simulink library "Fil"  (R2013b)
settings: Solver=ode45  StartTime=0.0  StopTime=10.0  RelTol=1e-3
libraries: Fil x5
settings Model: Creator=qzwc4r  LastModifiedBy=DZ1YRM

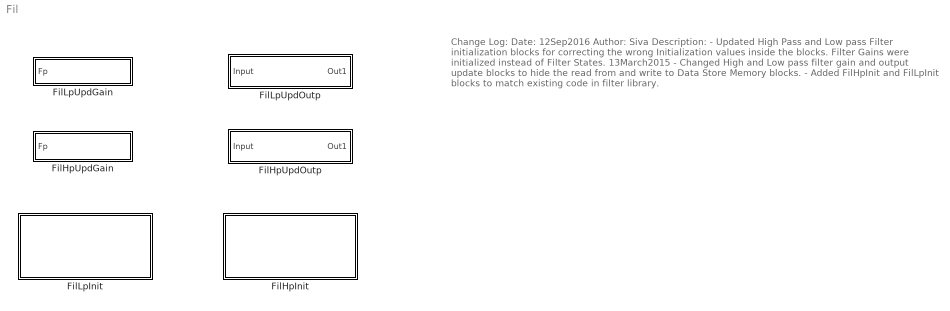
== system Fil ==
  note: Change Log:
      |
      | Date: 12Sep2016
      | Author: Siva
      | Description:
      |      -  Updated High Pass and Low pass Filter initialization blocks for correcting the wrong Initialization values inside the blocks. Filter Gains were initialized instead of Filter States.
      |
      | 13March2015
      | - Changed High and Low pass filter gain and output update blocks to hide the read from and write to
      | Data Store Memory blocks.
      | - Added FilHpInit and FilLpInit blocks to match existing code in filter library.
  FilHpInit : Subsystem  mask(FilHpInit){Ic=0, Ts=0, Freq=0, StVar=DefaultValue}
      mask prompts: Ic "Initial Value"; Ts "TimeStep:"; Freq "Frequency:"; StVar "State Variable"
      mask init:
      | blk = gcb;
      | set_param([ blk '/FilHpUpdGain'],'StVar',StVar)
      | set_param([ blk '/FilHpUpdGain'],'Ts',Ts)
      | set_param([ blk '/FilLpInit'],'Ts',Ts)
      | set_param([ blk '/FilLpInit'],'Ic',Ic)
      | set_param([ blk '/FilLpInit'],'Freq',Freq)
      | set_param([ blk '/FilLpInit'],'StVar',StVar)
      | set_param([ blk '/Freq'],'Value',Freq)
      mask Display:
      | text(0.35,0.9,'FilHpInit')
      | text(0.05,0.7,['Ic: ' Ic])
      | text(0.05,0.5,['Ts: ' Ts])
      | text(0.05,0.3,['Freq: ' Freq])
      | text(0.05,0.1,['StVar: ' StVar])
  FilHpUpdGain : Subsystem  mask(FilHpUpdGain){Ts=0, StVar=DefaultValue}
      mask prompts: Ts "Time Step"; StVar "State Variable"
      mask help: Simulink implementation of the HPF_KUpdate_f32_m macro.
      mask init:
      | blk = gcb;
      | set_param([ blk '/FilLpUpdGain'],'StVar',StVar)
      | set_param([ blk '/Data Store Write'],'DataStoreName',StVar)
      | set_param([ blk '/Data Store Write'],'DataStoreElements',[StVar '.CorrnFac'])
      | set_param([ blk '/FilLpUpdGain'],'Ts',Ts)
      | set_param([ blk '/Constant5'],'Value',Ts)
      | set_param([ blk '/Constant4'],'Value',Ts)
      settings: AttributesFormatString=|
      | Ts: %<Ts>
      | StVar: %<StVar>
      mask Display:
      | port_label('input',1,'Hz');
      | text(0.25,0.5,'FilHpUpdGain')
  FilHpUpdOutp : Subsystem  mask(FilHpUpdOutp){StVar=DefaultValue}
      mask prompts: StVar "State Variable"
      mask help: Simulink implementation of the HPF_OpUpdate_f32_m macro.
      mask init:
      | blk = gcb;
      | set_param([ blk '/FilLpUpdOutp'],'StVar',StVar)
      | set_param([ blk '/Data Store Read'],'DataStoreName',StVar)
      | set_param([ blk '/Data Store Read'],'DataStoreElements',[StVar '.CorrnFac'])
      | set_param([ blk '/Data Store Write'],'DataStoreName',StVar)
      | set_param([ blk '/Data Store Write'],'DataStoreElements',[StVar '.FilLpRec.FilSt'])
      settings: AttributesFormatString=StVar: %<StVar>
      mask Display:
      | port_label('input',1,'Inp')
      | port_label('output',1,'Outp')
      | text(0.2,0.8,'FilHpUpdOutp')
  FilLpInit : Subsystem  mask(FilLpInit){Ic=0, Ts=0, Freq=0, StVar=DefaultValue}
      mask prompts: Ic "Initial Value"; Ts "TimeStep:"; Freq "Frequency:"; StVar "State Variable"
      mask init:
      | blk = gcb;
      | set_param([blk '/FilLpUpdGain'],'Ts',Ts)
      | set_param([blk '/FilLpUpdGain'],'StVar',StVar)
      | set_param([blk '/Freq'],'Value',Freq)
      | set_param([blk '/Ic'],'Value',Ic)
      | set_param([ blk '/Data Store Write'],'DataStoreName',StVar)
      | try
      |     dt = evalin('base',[StVar '.EngDT']);
      | catch err
      |     if strcmp(err.identifier,'MATLAB:undefinedVarOrClass')
      |         dt = struct.FilLpRec1;
      |     end
      | end
      | if isa(dt,'struct.FilLpRec1')
      | set_param([ blk '/Data Store Write'],'DataStoreElements',[StVar '.FilSt'])
      | elseif isa(dt,'struct.FilHpRec1')
      | set_param([ blk '/Data Store Write'],'DataStoreElements',[StVar '.FilLpRec.FilSt'])
      | else
      |     error('Incorrect data class.');
      | end
      mask Display:
      | text(0.35,0.9,'FilLpInit')
      | text(0.05,0.7,['Ic: ' Ic])
      | text(0.05,0.5,['Ts: ' Ts])
      | text(0.05,0.3,['Freq: ' Freq])
      | text(0.05,0.1,['StVar: ' StVar])
  FilLpUpdGain : Subsystem  mask(FilLpUpdGain){Ts=0, StVar=DefaulValue}
      mask prompts: Ts "Time Step:"; StVar "State Variable:"
      mask help: Simulink implementation of the LPF_KUpdate_f32_m macro.
      mask init:
      | blk = gcb;
      | set_param(blk,'StVar',StVar);
      | set_param([blk '/Data Store Write'],'DataStoreName',StVar);
      | set_param([blk '/Constant1'],'Value',Ts);
      | try
      |     dt = evalin('base',[StVar '.EngDT']);
      | catch err
      |     if strcmp(err.identifier,'MATLAB:undefinedVarOrClass')
      |         dt = struct.FilLpRec1;
      |     end
      | end
      | if isa(dt,'struct.FilLpRec1')
      | 
      | set_param([ blk '/Data Store Write'],'DataStoreElements',[StVar '.FilGain'])
      | elseif isa(dt,'struct.FilHpRec1')
      | set_param([ blk '/Data Store Write'],'DataStoreElements',[StVar '.FilLpRec.FilGain'])
      | else
      |     error('Incorrect data class.');
      | end
      settings: AttributesFormatString=|
      | Ts: %<Ts>
      | StVar: %<StVar>
      mask Display:
      | port_label('input',1,'Hz');
      | text(0.25,0.5,'FilLpUpdGain')
  FilLpUpdOutp : Subsystem  mask(FilLpUpdOutp){StVar=DefaulValue}
      mask prompts: StVar "State Variable:"
      mask help: Simulink implementation of the LPF_OpUpdate_f32_m macro.
      mask init:
      | blk = gcb;
      | set_param(blk,'StVar',StVar)
      | set_param([ blk '/Data Store Read'],'DataStoreName',StVar)
      | set_param([ blk '/Data Store Write'],'DataStoreName',StVar)
      | try
      |     dt = evalin('base',[StVar '.EngDT']);
      | catch err
      |     if strcmp(err.identifier,'MATLAB:undefinedVarOrClass')
      |         dt = struct.FilLpRec1;
      |     end
      | end
      | if isa(dt,'struct.FilLpRec1')
      | set_param([ blk '/Data Store Read'],'DataStoreElements',[StVar '.FilSt#' StVar '.FilGain'])
      | set_param([ blk '/Data Store Write'],'DataStoreElements',[StVar '.FilSt'])
      | elseif isa(dt,'struct.FilHpRec1')
      | set_param([ blk '/Data Store Read'],'DataStoreElements',[StVar '.FilLpRec.FilSt#' StVar '.FilLpRec.FilGain'])
      | set_param([ blk '/Data Store Write'],'DataStoreElements',[StVar '.FilLpRec.FilSt'])
      | else
      |     error('Incorrect data class.');
      | end
      settings: AttributesFormatString=StVar: %<StVar>
      mask Display:
      | port_label('input',1,'Inp')
      | port_label('output',1,'Outp')
      | text(0.2,0.8,'FilLpUpdOutp')

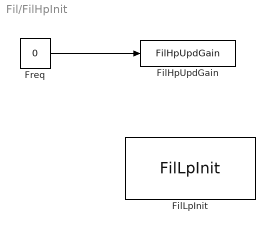
== system Fil/FilHpInit ==
  FilHpUpdGain : Fil/FilHpUpdGain  Ts=0  StVar=DefaultValue
      settings: AttributesFormatString=|
      | Ts: %<Ts>
      | StVar: %<StVar>
  FilLpInit : Fil/FilLpInit  Ic=0  Ts=0  Freq=0  StVar=DefaultValue
  Freq : Constant  Value=0  OutDataTypeStr=single
  wires:
  Freq/1 -> FilHpUpdGain/1

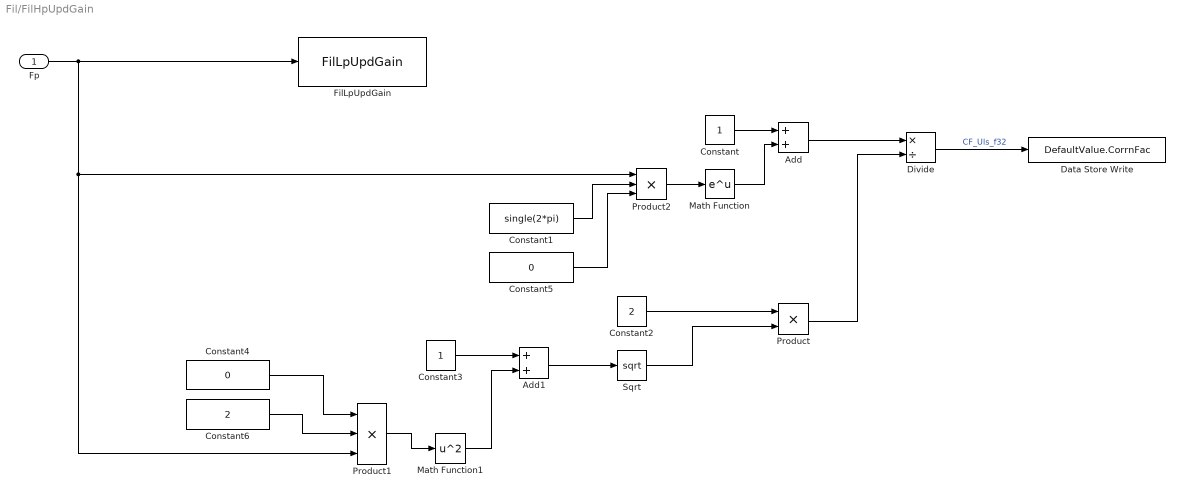
== system Fil/FilHpUpdGain ==
  Fp : Inport
  Add : Sum
  Add1 : Sum
  Constant : Constant  OutDataTypeStr=single
  Constant1 : Constant  Value=single(2*pi)  OutDataTypeStr=single
  Constant2 : Constant  Value=2  OutDataTypeStr=single
  Constant3 : Constant  OutDataTypeStr=single
  Constant4 : Constant  Value=0  OutDataTypeStr=single
  Constant5 : Constant  Value=0  OutDataTypeStr=single
  Constant6 : Constant  Value=2  OutDataTypeStr=single
  Data Store Write : DataStoreWrite  DataStoreName=DefaultValue  DataStoreElements=DefaultValue.CorrnFac
  Divide : Product  Inputs=*/
  FilLpUpdGain : Fil/FilLpUpdGain  Ts=0  StVar=DefaultValue
      settings: AttributesFormatString=|
      | StVar: %<StVar>
      | Time Step: %<Ts>
  Math Function : Math  SaturateOnIntegerOverflow=on
  Math Function1 : Math  Operator=square  SaturateOnIntegerOverflow=on
  Product : Product
  Product1 : Product  Inputs=3
  Product2 : Product  Inputs=3
  Sqrt : Sqrt  SaturateOnIntegerOverflow=on
  wires:
  Constant6/1 -> Product1/2
  Constant5/1 -> Product2/3
  Divide/1 -> Data Store Write/1  "CF_Uls_f32"
  Product1/1 -> Math Function1/1
  Math Function1/1 -> Add1/2
  Product2/1 -> Math Function/1
  Product/1 -> Divide/2
  Constant4/1 -> Product1/1
  Add1/1 -> Sqrt/1
  Constant3/1 -> Add1/1
  Constant2/1 -> Product/1
  Sqrt/1 -> Product/2
  Add/1 -> Divide/1
  Math Function/1 -> Add/2
  Constant1/1 -> Product2/2
  Constant/1 -> Add/1
  Fp/1 -> FilLpUpdGain/1, Product2/1, Product1/3

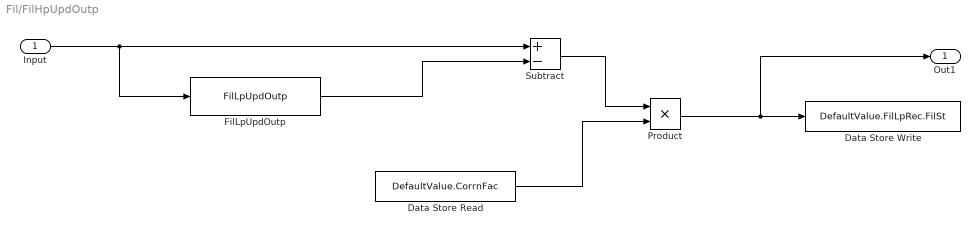
== system Fil/FilHpUpdOutp ==
  Input : Inport
  Data Store Read : DataStoreRead  DataStoreName=DefaultValue  DataStoreElements=DefaultValue.CorrnFac
  Data Store Write : DataStoreWrite  DataStoreName=DefaultValue  DataStoreElements=DefaultValue.FilLpRec.FilSt
  FilLpUpdOutp : Fil/FilLpUpdOutp  StVar=DefaultValue
  Product : Product
  Subtract : Sum  Inputs=+-
  Out1 : Outport
  wires:
  Product/1 -> Out1/1, Data Store Write/1
  Subtract/1 -> Product/1
  Input/1 -> FilLpUpdOutp/1, Subtract/1
  FilLpUpdOutp/1 -> Subtract/2
  Data Store Read/1 -> Product/2

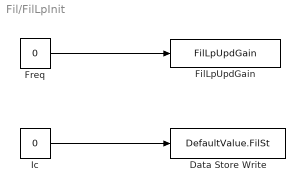
== system Fil/FilLpInit ==
  Data Store Write : DataStoreWrite  DataStoreName=DefaultValue  DataStoreElements=DefaultValue.FilSt
  FilLpUpdGain : Fil/FilLpUpdGain  Ts=0  StVar=DefaultValue
  Freq : Constant  Value=0  OutDataTypeStr=single
  Ic : Constant  Value=0  OutDataTypeStr=single
  wires:
  Freq/1 -> FilLpUpdGain/1
  Ic/1 -> Data Store Write/1

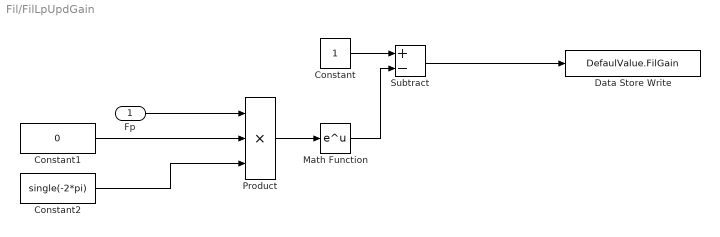
== system Fil/FilLpUpdGain ==
  Fp : Inport  OutDataTypeStr=single
  Constant : Constant  OutDataTypeStr=single
  Constant1 : Constant  Value=0  OutDataTypeStr=single
  Constant2 : Constant  Value=single(-2*pi)  OutDataTypeStr=single
  Data Store Write : DataStoreWrite  DataStoreName=DefaulValue  DataStoreElements=DefaulValue.FilGain
  Math Function : Math  SaturateOnIntegerOverflow=on
  Product : Product  Inputs=3
  Subtract : Sum  Inputs=+-
  wires:
  Constant2/1 -> Product/3
  Product/1 -> Math Function/1
  Fp/1 -> Product/1
  Constant1/1 -> Product/2
  Math Function/1 -> Subtract/2
  Constant/1 -> Subtract/1
  Subtract/1 -> Data Store Write/1

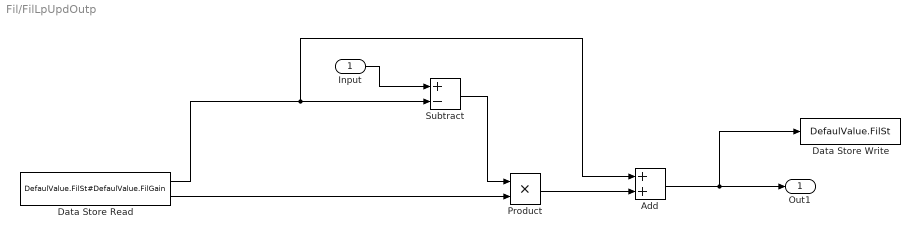
== system Fil/FilLpUpdOutp ==
  Input : Inport
  Add : Sum
  Data Store Read : DataStoreRead  DataStoreName=DefaulValue  DataStoreElements=DefaulValue.FilSt#DefaulValue.FilGain
  Data Store Write : DataStoreWrite  DataStoreName=DefaulValue  DataStoreElements=DefaulValue.FilSt
  Product : Product
  Subtract : Sum  Inputs=+-
  Out1 : Outport  OutDataTypeStr=single
  wires:
  Data Store Read/1 -> Add/1, Subtract/2
  Input/1 -> Subtract/1
  Subtract/1 -> Product/1
  Product/1 -> Add/2
  Add/1 -> Data Store Write/1, Out1/1
  Data Store Read/2 -> Product/2
